simulink model "PMSM_My_PI"  (R2017b)
settings: Solver=VariableStepAuto  StartTime=0.0  StopTime=0.2  FixedStep=0.000001  MaxStep=1e-4  RelTol=1e-3
undefined symbols (not defined in the file or in its folder): sigbuilder_block
libraries: powerlib x21, simulink x1
settings Model: Creator=Linyc  LastModifiedBy=Crazyyiwen

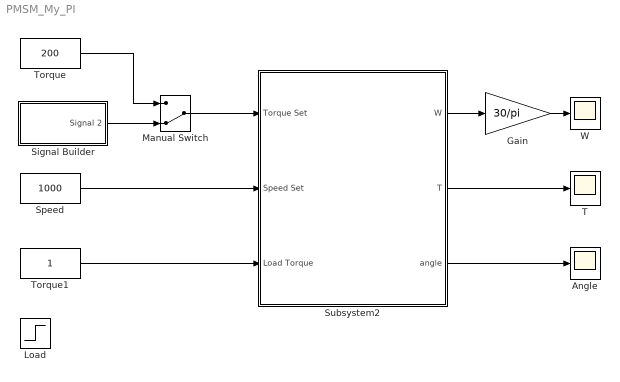
== system PMSM_My_PI ==
  Angle : Scope
  Gain : Gain  Gain=30/pi
  Load : Step  Time=0.02  After=0  SampleTime=0
  Manual Switch : ManualSwitch  CurrentSetting=0
  Signal Builder : Subsystem  Tag=STV Subsys  LoadFcn=sigbuilder_block('load');  StartFcn=sigbuilder_block('start');  StopFcn=sigbuilder_block('stop');  ClipboardFcn=sigbuilder_block('clipboard');  mask(Sigbuilder block){tuvar=[0:10]}
      mask help: Simulink:masks:SigbuilderBlock_MD
      mask init:
      | if ~strcmp(get_param(bdroot(gcbh),'SimulationStatus'),'stopped') tuvar = sigbuilder_block('maskInit'); end
      settings: CopyFcn=sigbuilder_block('copy');  DeleteFcn=sigbuilder_block('delete');  ModelCloseFcn=sigbuilder_block('modelClose');  PreSaveFcn=sigbuilder_block('preSave');  PauseFcn=sigbuilder_block('pause');  ContinueFcn=sigbuilder_block('continue');  NameChangeFcn=sigbuilder_block('namechange');  OpenFcn=sigbuilder_block('open',[424.5 166.5 847.5 399.75 ]);  CloseFcn=sigbuilder_block('close');
      mask Display: plot(0, 0, 100, 100,[2, 2, 32, 32, 2], [68, 8, 8, 68, 68],[32, 2], [38, 38], [32, 19, 2],[53, 60, 44], [32, 17, 17, 2],[16, 16, 31, 31]);txt = getActiveGroup(gcbh);text(2, 100, txt,'verticalAlignment', 'top');
  Speed : Constant  Value=1000
  Subsystem2 : Subsystem
  T : Scope
  Torque : Constant  Value=200
  Torque1 : Constant
  W : Scope
  wires:
  Speed/1 -> Subsystem2/2(Speed Set)
  Subsystem2/1(W) -> Gain/1
  Subsystem2/2(T) -> T/1
  Subsystem2/3(angle) -> Angle/1
  Gain/1 -> W/1
  Torque/1 -> Manual Switch/1
  Manual Switch/1 -> Subsystem2/1(Torque Set)
  Signal Builder/1(Signal 2) -> Manual Switch/2
  Torque1/1 -> Subsystem2/3(Load Torque)

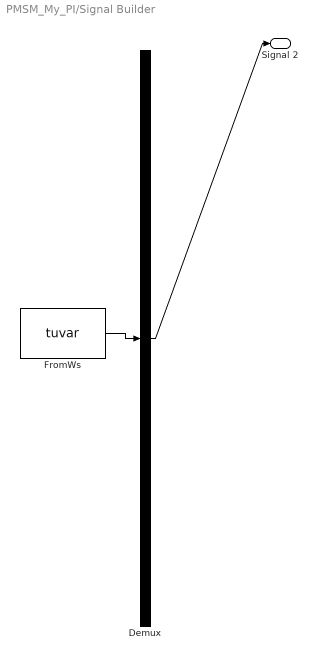
== system PMSM_My_PI/Signal Builder ==
  Demux : Demux  Tag=STV Demux  Outputs=1
  FromWs : FromWorkspace  Tag=STV FromWs  VariableName=tuvar  SampleTime=0
      SigBuilderData=|
      | common.afterFinalStr = 'Extrapolate'
      | common.sampleTime = 0
      | dataSet.timeRange = [0 2]
      | dataSet.name = 'Group 1'
      | sbobj.Groups.Name = 'Group 1'
      | sbobj.Groups.Signals.Name = 'Signal 2'
      | sbobj.Groups.Signals.XData = [0 1 1 2]
      | sbobj.Groups.Signals.YData = [200 200 0 0]
      | sbobj.Groups.TimeRange = [0 2]
  Signal 2 : Outport  Tag=STV Outport
  wires:
  FromWs/1 -> Demux/1
  Demux/1 -> Signal 2/1

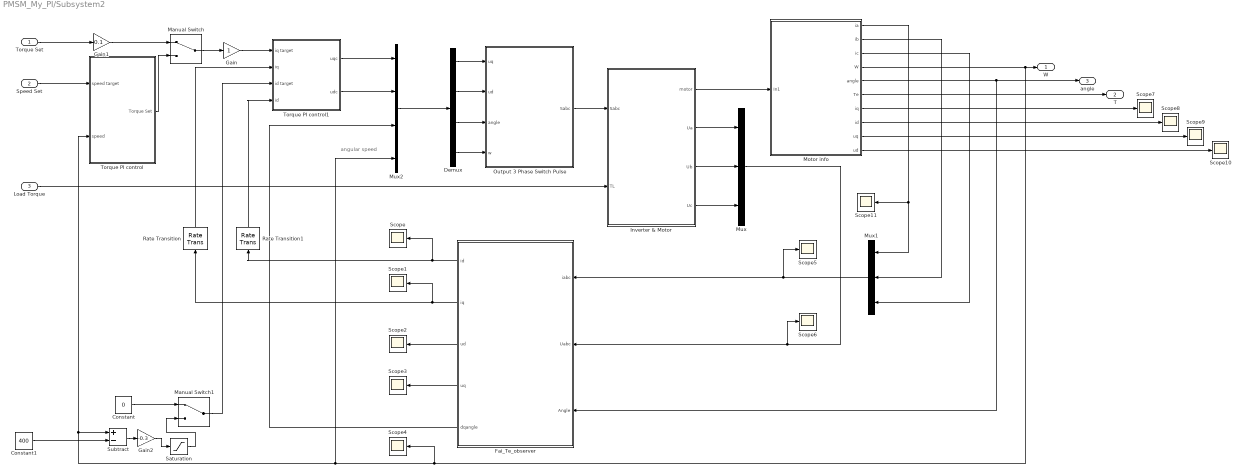
== system PMSM_My_PI/Subsystem2 ==
  note: angular speed
  Torque Set : Inport
  Speed Set : Inport  Port=2
  Load Torque : Inport  Port=3
  Constant : Constant  Value=0
  Constant1 : Constant  Value=400
  Demux : Demux
  Fai_Te_observer : Subsystem
  Gain : Gain
  Gain1 : Gain  Gain=0.1
  Gain2 : Gain  Gain=-0.3
  Inverter & Motor : Subsystem
  Manual Switch : ManualSwitch
  Manual Switch1 : ManualSwitch
  Motor info : Subsystem
  Mux : Mux  Inputs=3
  Mux1 : Mux  Inputs=3
  Mux2 : Mux
  Output 3 Phase Switch Pulse : Subsystem
  Rate Transition : RateTransition  OutPortSampleTime=0.0002
  Rate Transition1 : RateTransition  OutPortSampleTime=0.0002
  Saturation : Saturate  UpperLimit=0  LowerLimit=-150
  Scope{,1..11} (12 alike) : Scope
  Subtract : Sum  Inputs=+-
  Torque PI control : Subsystem
  Torque PI control1 : Subsystem
  W : Outport
  T : Outport  Port=2
  angle : Outport  Port=3
  wires:
  Motor info/4(W) -> Scope4/1, Mux2/4, Subtract/1, Torque PI control/2(speed), W/1
  Load Torque/1 -> Inverter & Motor/2(TL)
  Motor info/6(Te) -> T/1
  Inverter & Motor/1(motor) -> Motor info/1(In1)
  Motor info/5(angle) -> Fai_Te_observer/3(Angle), angle/1
  Motor info/1(ia) -> Scope11/1, Mux1/1
  Motor info/2(ib) -> Mux1/2
  Motor info/3(ic) -> Mux1/3
  Output 3 Phase Switch Pulse/1(Sabc) -> Inverter & Motor/1(Sabc)
  Mux1/1 -> Fai_Te_observer/1(iabc), Scope5/1
  Mux/1 -> Fai_Te_observer/2(Uabc), Scope6/1
  Mux2/1 -> Demux/1
  Motor info/7(iq) -> Scope7/1
  Motor info/8(id) -> Scope8/1
  Motor info/9(uq) -> Scope9/1
  Motor info/10(ud) -> Scope10/1
  Fai_Te_observer/1(id) -> Rate Transition1/1, Scope/1
  Fai_Te_observer/2(iq) -> Rate Transition/1, Scope1/1
  Fai_Te_observer/3(ud) -> Scope2/1
  Fai_Te_observer/4(uq) -> Scope3/1
  Speed Set/1 -> Torque PI control/1(speed target)
  Torque Set/1 -> Gain1/1
  Torque PI control/1(Torque Set) -> Manual Switch/2
  Fai_Te_observer/5(dqangle) -> Mux2/3
  Manual Switch/1 -> Gain/1
  Gain/1 -> Torque PI control1/1(iq target)
  Demux/1 -> Output 3 Phase Switch Pulse/1(uq)
  Demux/2 -> Output 3 Phase Switch Pulse/2(ud)
  Demux/3 -> Output 3 Phase Switch Pulse/3(angle)
  Torque PI control1/1(uqc) -> Mux2/1
  Rate Transition/1 -> Torque PI control1/2(iq)
  Demux/4 -> Output 3 Phase Switch Pulse/4(w)
  Gain1/1 -> Manual Switch/1
  Torque PI control1/2(udc) -> Mux2/2
  Rate Transition1/1 -> Torque PI control1/4(id)
  Constant/1 -> Manual Switch1/1
  Manual Switch1/1 -> Torque PI control1/3(id target)
  Constant1/1 -> Subtract/2
  Subtract/1 -> Gain2/1
  Gain2/1 -> Saturation/1
  Saturation/1 -> Manual Switch1/2
  Inverter & Motor/2(Ua) -> Mux/1
  Inverter & Motor/3(Ub) -> Mux/2
  Inverter & Motor/4(Uc) -> Mux/3

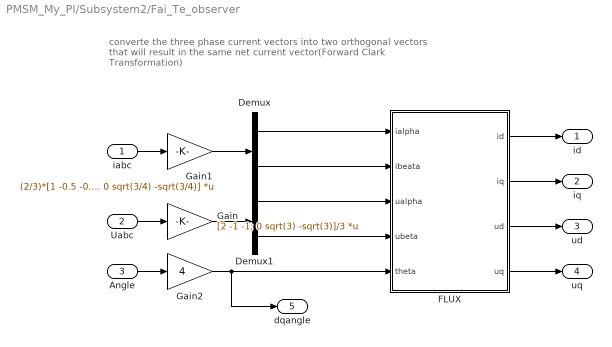
== system PMSM_My_PI/Subsystem2/Fai_Te_observer ==
  note: converte the three phase current vectors into
      | two orthogonal vectors that will result in the
      | same net current vector(Forward Clark Transformation)
  iabc : Inport
  Uabc : Inport  Port=2
  Angle : Inport  Port=3
  Demux : Demux  Outputs=2
  Demux1 : Demux  Outputs=2
  FLUX : Subsystem
  Gain : Gain  Gain=[2 -1 -1; 0 sqrt(3) -sqrt(3)]/3  Multiplication=Matrix(K*u)
  Gain1 : Gain  Gain=(2/3)*[1 -0.5 -0.5; 0 sqrt(3/4) -sqrt(3/4)]  Multiplication=Matrix(K*u)
  Gain2 : Gain  Gain=4
  id : Outport
  iq : Outport  Port=2
  ud : Outport  Port=3
  uq : Outport  Port=4
  dqangle : Outport  Port=5
  wires:
  Demux/1 -> FLUX/1(ialpha)
  Gain/1 -> Demux1/1
  iabc/1 -> Gain1/1
  Demux/2 -> FLUX/2(ibeata)
  Demux1/2 -> FLUX/4(ubeta)
  Demux1/1 -> FLUX/3(ualpha)
  Uabc/1 -> Gain/1
  Gain1/1 -> Demux/1
  Angle/1 -> Gain2/1
  Gain2/1 -> dqangle/1, FLUX/5(theta)
  FLUX/1(id) -> id/1
  FLUX/2(iq) -> iq/1
  FLUX/3(ud) -> ud/1
  FLUX/4(uq) -> uq/1

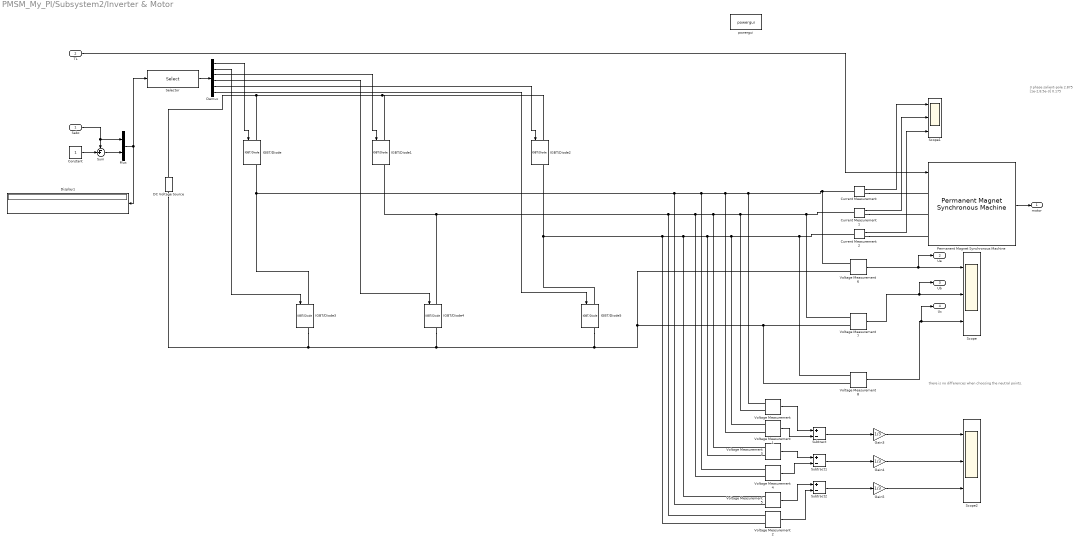
== system PMSM_My_PI/Subsystem2/Inverter & Motor ==
  note: there is no differences when choosing the neutral points.
  note: 3 phase
      | salient-pole
      |
      | 2.875
      | [1e-2,8.5e-3]
      | 0.175
  Sabc : Inport
  TL : Inport  Port=2
  Constant : Constant
  Current Measurement : powerlib/Measurements/Current Measurement  PhasorSimulation=off  OutputType=Complex  PSBequivalent=0
  Current Measurement1 : powerlib/Measurements/Current Measurement  PhasorSimulation=off  OutputType=Complex  PSBequivalent=0
  Current Measurement2 : powerlib/Measurements/Current Measurement  PhasorSimulation=off  OutputType=Complex  PSBequivalent=0
  DC Voltage Source : powerlib/Electrical Sources/DC Voltage Source  Amplitude=380  Measurements=None
  Demux : Demux  Outputs=6
  Display1 : Display
  Gain3 : Gain  Gain=1/3
  Gain4 : Gain  Gain=1/3
  Gain5 : Gain  Gain=1/3
  IGBT/Diode{,1..5} (6 alike) : powerlib/Power Electronics/IGBT//Diode  Ron=1e-2  Rs=1e4  Cs=inf  Measurements=on
  Mux : Mux  Inputs=2
  Permanent Magnet Synchronous Machine : powerlib/Machines/Permanent Magnet Synchronous Machine  NbPhases=3  FluxDistribution=Sinusoidal  RotorType=Salient-pole  MechanicalLoad=Torque Tm  PresetModel=No  ShowDetailedParameters=on  MeasurementBus=off  Resistance=2.875  Inductance=8.5e-3  dqInductances=[1e-2,8.5e-3]  La=0.000395  MachineConstant=Flux linkage established by magnets (V.s)  Flux=0.175  VoltageCst=126.966  TorqueCst=1.05  Flat=120  Mechanical=[0.0027 0.175 4 0]  PolePairs=2  InitialConditions=[0,0, 0,0]  InitialConditions5ph=[0 0 0 0 0 0]  TsPowergui=0  TsBlock=-1  RefAngle=Aligned with phase A axis (original Park)
      settings: SourceProductName=Simscape Power Systems
  Scope : Scope  NumInputPorts=3
  Scope1 : Scope  NumInputPorts=3
  Scope2 : Scope  NumInputPorts=3
  Selector : Selector  InputPortWidth=6  IndexOptions=Index vector (dialog)  Indices=[1 4 2 5 3 6]  OutputSizes=1
  Subtract : Sum  Inputs=+-
  Subtract1 : Sum  Inputs=+-
  Subtract2 : Sum  Inputs=+-
  Sum : Sum  Inputs=-+|
  Voltage Measurement{,1..8} (9 alike) : powerlib/Measurements/Voltage Measurement  PhasorSimulation=off  OutputType=Complex  PSBequivalent=0
  powergui : powerlib/powergui  Priority=1  SimulationMode=Continuous  SampleTime=0.000001  frequency=60  Iterations=50  frequencyindice=0  Pbase=100e6  ErrMax=1e-4  UnitsV=kV  UnitsW=MW  buscounter=0  FunctionMessages=on  echomessages=off  EnableUseOfTLC=off  CurrentSourceSwitches=off  DisableSnubberDevices=off  DisableRonSwitches=off  DisableVfSwitches=off  DisplayEquations=off  SolverType=Tustin/Backward Euler (TBE)  Interpol=off  ExternalGateDelay=off  methode=off  Ts=100  x0status=blocks  SPID=on  SwTol=0  HookPort=off  RestoreLinks=warning  ResistiveCurrentMeasurement=off  Frange=[0:2:500]  Ylog=off  Xlog=on  ShowGrid=off  save=off  variable=ZData  structure=0  ZoomFFT=off  StartTime=0.0  cycles=1  DisplayStyle=1  fundamental=60  FreqAxis=off  MaxFrequency=1000  frequencyindicesteady=1  RmsSteady=1  display=off
  motor : Outport
  Ua : Outport  Port=2
  Ub : Outport  Port=3
  Uc : Outport  Port=4
  wires:
  Constant/1 -> Sum/2
  Sum/1 -> Mux/2
  Mux/1 -> Display1/1, Selector/1
  TL/1 -> Permanent Magnet Synchronous Machine/1
  Permanent Magnet Synchronous Machine/1 -> motor/1
  Sabc/1 -> Mux/1, Sum/1
  Selector/1 -> Demux/1
  Demux/1 -> IGBT/Diode/1
  Demux/2 -> IGBT/Diode3/1
  Demux/3 -> IGBT/Diode1/1
  Demux/4 -> IGBT/Diode4/1
  Demux/5 -> IGBT/Diode2/1
  Demux/6 -> IGBT/Diode5/1
  Voltage Measurement7/1 -> Ub/1, Scope/2
  Voltage Measurement6/1 -> Ua/1, Scope/1
  Voltage Measurement8/1 -> Uc/1, Scope/3
  Current Measurement/1 -> Scope1/1
  Current Measurement1/1 -> Scope1/2
  Current Measurement2/1 -> Scope1/3
  Gain3/1 -> Scope2/1
  Gain4/1 -> Scope2/2
  Gain5/1 -> Scope2/3
  Voltage Measurement/1 -> Subtract/1
  Voltage Measurement1/1 -> Subtract/2
  Voltage Measurement3/1 -> Subtract1/1
  Voltage Measurement4/1 -> Subtract1/2
  Voltage Measurement5/1 -> Subtract2/1
  Voltage Measurement2/1 -> Subtract2/2
  Subtract/1 -> Gain3/1
  Subtract1/1 -> Gain4/1
  Subtract2/1 -> Gain5/1
  connections:
  IGBT/Diode/RConn1 -- Voltage Measurement5/LConn2 -- Voltage Measurement4/LConn1 -- Voltage Measurement1/LConn2 -- Voltage Measurement/LConn1 -- Voltage Measurement6/LConn1 -- Current Measurement/LConn1 -- IGBT/Diode3/LConn1
  DC Voltage Source/RConn1 -- IGBT/Diode2/LConn1 -- IGBT/Diode1/LConn1 -- IGBT/Diode/LConn1
  IGBT/Diode1/RConn1 -- Voltage Measurement2/LConn1 -- Voltage Measurement4/LConn2 -- Voltage Measurement3/LConn1 -- Voltage Measurement/LConn2 -- Voltage Measurement7/LConn1 -- Current Measurement1/LConn1 -- IGBT/Diode4/LConn1
  IGBT/Diode2/RConn1 -- Voltage Measurement2/LConn2 -- Voltage Measurement5/LConn1 -- Voltage Measurement3/LConn2 -- Voltage Measurement1/LConn1 -- Voltage Measurement8/LConn1 -- Current Measurement2/LConn1 -- IGBT/Diode5/LConn1
  IGBT/Diode5/RConn1 -- Voltage Measurement8/LConn2 -- Voltage Measurement7/LConn2 -- Voltage Measurement6/LConn2 -- DC Voltage Source/LConn1 -- IGBT/Diode3/RConn1 -- IGBT/Diode4/RConn1
  Current Measurement/RConn1 -- Permanent Magnet Synchronous Machine/LConn1
  Current Measurement1/RConn1 -- Permanent Magnet Synchronous Machine/LConn2
  Current Measurement2/RConn1 -- Permanent Magnet Synchronous Machine/LConn3

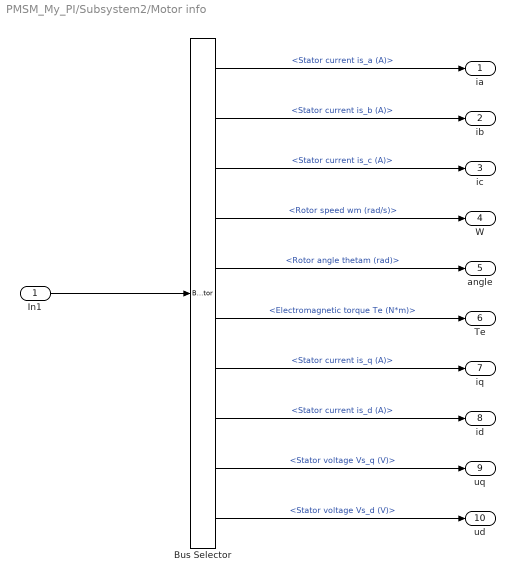
== system PMSM_My_PI/Subsystem2/Motor info ==
  In1 : Inport
  Bus Selector : BusSelector  OutputSignals=Stator current is_a (A),Stator current is_b (A),Stator current is_c (A),Rotor speed wm (rad/s),Rotor angle thetam (rad),Electromagnetic torque Te (N*m),Stator current is_q (A),Stator current is_d (A),Stator voltage Vs_q (V),Stator voltage Vs_d (V)
  ia : Outport
  ib : Outport  Port=2
  ic : Outport  Port=3
  W : Outport  Port=4
  angle : Outport  Port=5
  Te : Outport  Port=6
  iq : Outport  Port=7
  id : Outport  Port=8
  uq : Outport  Port=9
  ud : Outport  Port=10
  wires:
  In1/1 -> Bus Selector/1
  Bus Selector/2 -> ib/1  "<Stator current is_b (A)>"
  Bus Selector/3 -> ic/1  "<Stator current is_c (A)>"
  Bus Selector/6 -> Te/1  "<Electromagnetic torque Te (N*m)>"
  Bus Selector/1 -> ia/1  "<Stator current is_a (A)>"
  Bus Selector/5 -> angle/1  "<Rotor angle thetam (rad)>"
  Bus Selector/4 -> W/1  "<Rotor speed wm (rad/s)>"
  Bus Selector/7 -> iq/1  "<Stator current is_q (A)>"
  Bus Selector/8 -> id/1  "<Stator current is_d (A)>"
  Bus Selector/9 -> uq/1  "<Stator voltage Vs_q (V)>"
  Bus Selector/10 -> ud/1  "<Stator voltage Vs_d (V)>"

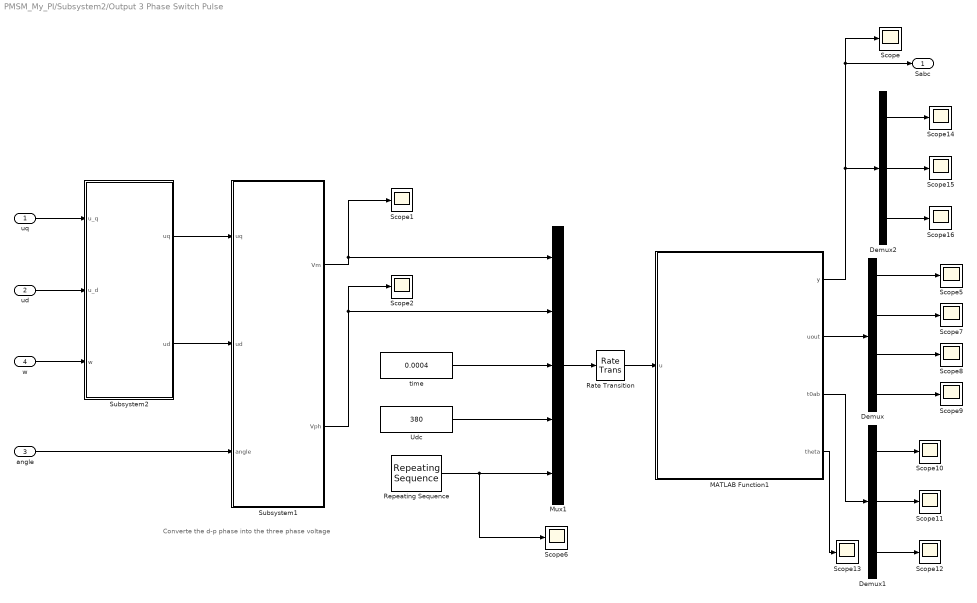
== system PMSM_My_PI/Subsystem2/Output 3 Phase Switch Pulse ==
  note: Converte the d-p phase into the three phase voltage
  uq : Inport
  ud : Inport  Port=2
  angle : Inport  Port=3
  w : Inport  Port=4
  Demux : Demux
  Demux1 : Demux  Outputs=3
  Demux2 : Demux  Outputs=3
  MATLAB Function1 : MATLAB Function  TreatAsAtomicUnit=on
  Mux1 : Mux  Inputs=5
  Rate Transition : RateTransition  OutPortSampleTime=0.000001
  Repeating Sequence : simulink/Sources/Repeating Sequence  rep_seq_t=[0 0.0002 0.0004]  rep_seq_y=[0 380 0]
  Scope{,1..2,5..16} (15 alike) : Scope
  Subsystem1 : Subsystem
  Subsystem2 : Subsystem
  Udc : Constant  Value=380
  time : Constant  Value=0.0004
  Sabc : Outport
  wires:
  time/1 -> Mux1/3
  Repeating Sequence/1 -> Scope6/1, Mux1/5
  Udc/1 -> Mux1/4
  MATLAB Function1/1(y) -> Demux2/1, Scope/1, Sabc/1
  Subsystem1/1(Vm) -> Mux1/1, Scope1/1
  Subsystem1/2(Vph) -> Mux1/2, Scope2/1
  Mux1/1 -> Rate Transition/1
  MATLAB Function1/2(uout) -> Demux/1
  Demux/4 -> Scope9/1
  Demux/2 -> Scope7/1
  Demux/3 -> Scope8/1
  Demux/1 -> Scope5/1
  MATLAB Function1/3(t0ab) -> Demux1/1
  Demux1/1 -> Scope10/1
  Demux1/3 -> Scope12/1
  Demux1/2 -> Scope11/1
  MATLAB Function1/4(theta) -> Scope13/1
  Demux2/2 -> Scope15/1
  Demux2/3 -> Scope16/1
  Demux2/1 -> Scope14/1
  Rate Transition/1 -> MATLAB Function1/1(u)
  uq/1 -> Subsystem2/1(u_q)
  ud/1 -> Subsystem2/2(u_d)
  Subsystem2/1(uq) -> Subsystem1/1(uq)
  Subsystem2/2(ud) -> Subsystem1/2(ud)
  angle/1 -> Subsystem1/3(angle)
  w/1 -> Subsystem2/3(w)

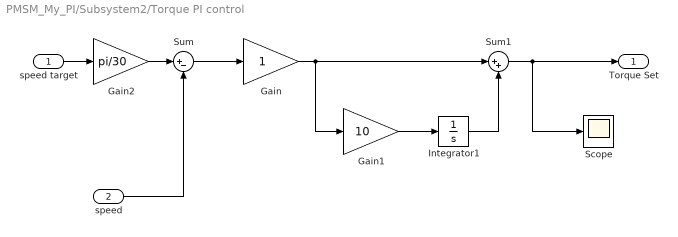
== system PMSM_My_PI/Subsystem2/Torque PI control ==
  speed target : Inport
  speed : Inport  Port=2
  Gain : Gain
  Gain1 : Gain  Gain=10
  Gain2 : Gain  Gain=pi/30
  Integrator1 : Integrator
  Scope : Scope
  Sum : Sum  Inputs=|+-
  Sum1 : Sum  Inputs=|++
  Torque Set : Outport
  wires:
  speed target/1 -> Gain2/1
  Sum/1 -> Gain/1
  speed/1 -> Sum/2
  Gain2/1 -> Sum/1
  Gain/1 -> Gain1/1, Sum1/1
  Integrator1/1 -> Sum1/2
  Sum1/1 -> Scope/1, Torque Set/1
  Gain1/1 -> Integrator1/1

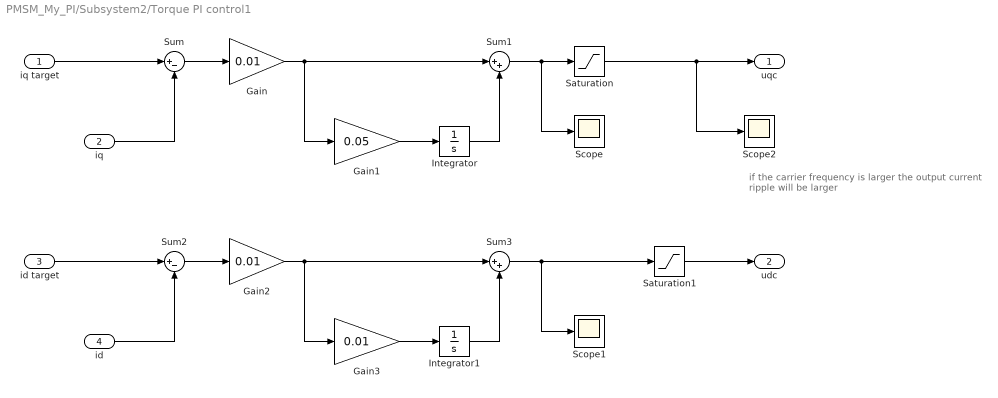
== system PMSM_My_PI/Subsystem2/Torque PI control1 ==
  note: if the carrier frequency is larger the
      | output current ripple will be larger
  iq target : Inport
  iq : Inport  Port=2
  id target : Inport  Port=3
  id : Inport  Port=4
  Gain : Gain  Gain=0.01
  Gain1 : Gain  Gain=0.05
  Gain2 : Gain  Gain=0.01
  Gain3 : Gain  Gain=0.01
  Integrator : Integrator
  Integrator1 : Integrator
  Saturation : Saturate  UpperLimit=1  LowerLimit=-1
  Saturation1 : Saturate  UpperLimit=1  LowerLimit=-1
  Scope : Scope
  Scope1 : Scope
  Scope2 : Scope
  Sum : Sum  Inputs=|+-
  Sum1 : Sum  Inputs=|++
  Sum2 : Sum  Inputs=|+-
  Sum3 : Sum  Inputs=|++
  uqc : Outport
  udc : Outport  Port=2
  wires:
  Gain1/1 -> Integrator/1
  Integrator/1 -> Sum1/2
  Gain/1 -> Gain1/1, Sum1/1
  iq/1 -> Sum/2
  Sum/1 -> Gain/1
  id target/1 -> Sum2/1
  Sum2/1 -> Gain2/1
  id/1 -> Sum2/2
  Gain2/1 -> Sum3/1, Gain3/1
  Sum3/1 -> Saturation1/1, Scope1/1
  Integrator1/1 -> Sum3/2
  Gain3/1 -> Integrator1/1
  Saturation1/1 -> udc/1
  iq target/1 -> Sum/1
  Sum1/1 -> Saturation/1, Scope/1
  Saturation/1 -> Scope2/1, uqc/1

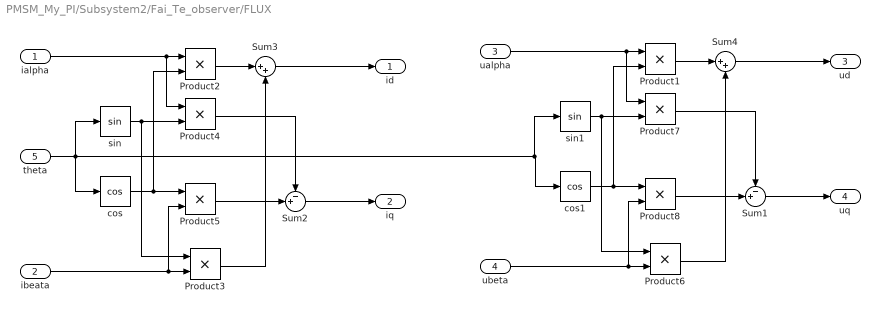
== system PMSM_My_PI/Subsystem2/Fai_Te_observer/FLUX ==
  ialpha : Inport
  ibeata : Inport  Port=2
  ualpha : Inport  Port=3
  ubeta : Inport  Port=4
  theta : Inport  Port=5
  Product{1..8} (8 alike) : Product
  Sum1 : Sum  Inputs=-+|
  Sum2 : Sum  Inputs=-+|
  Sum3 : Sum  Inputs=|++
  Sum4 : Sum  Inputs=|++
  cos : Trigonometry  Operator=cos
  cos1 : Trigonometry  Operator=cos
  sin : Trigonometry
  sin1 : Trigonometry
  id : Outport
  iq : Outport  Port=2
  ud : Outport  Port=3
  uq : Outport  Port=4
  wires:
  ialpha/1 -> Product4/1, Product2/1
  cos/1 -> Product5/1, Product2/2
  ibeata/1 -> Product5/2, Product3/2
  sin/1 -> Product4/2, Product3/1
  Product2/1 -> Sum3/1
  Product3/1 -> Sum3/2
  Product4/1 -> Sum2/1
  Product5/1 -> Sum2/2
  Sum3/1 -> id/1
  Sum2/1 -> iq/1
  Sum1/1 -> uq/1
  Sum4/1 -> ud/1
  Product8/1 -> Sum1/2
  Product7/1 -> Sum1/1
  Product6/1 -> Sum4/2
  Product1/1 -> Sum4/1
  sin1/1 -> Product6/1, Product7/2
  ubeta/1 -> Product6/2, Product8/2
  cos1/1 -> Product1/2, Product8/1
  ualpha/1 -> Product1/1, Product7/1
  theta/1 -> sin1/1, cos1/1, sin/1, cos/1

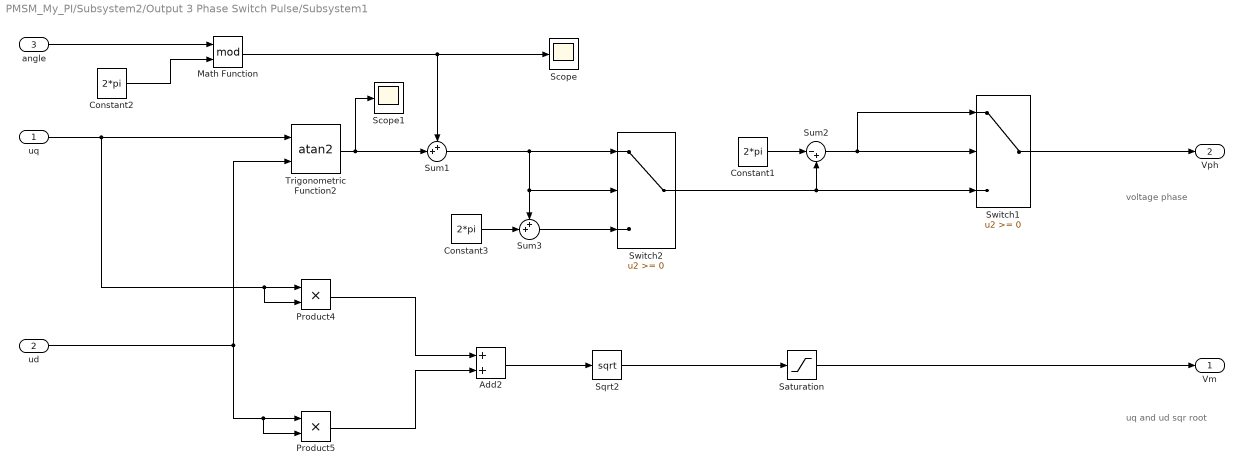
== system PMSM_My_PI/Subsystem2/Output 3 Phase Switch Pulse/Subsystem1 ==
  note: voltage phase
  note: uq and ud sqr root
  uq : Inport
  ud : Inport  Port=2
  angle : Inport  Port=3
  Add2 : Sum
  Constant1 : Constant  Value=2*pi
  Constant2 : Constant  Value=2*pi
  Constant3 : Constant  Value=2*pi
  Math Function : Math  Operator=mod  SaturateOnIntegerOverflow=on
  Product4 : Product
  Product5 : Product
  Saturation : Saturate  UpperLimit=380  LowerLimit=0
  Scope : Scope
  Scope1 : Scope
  Sqrt2 : Sqrt  SaturateOnIntegerOverflow=on
  Sum1 : Sum  Inputs=++|
  Sum2 : Sum  Inputs=|-+
  Sum3 : Sum  Inputs=++|
  Switch1 : Switch
  Switch2 : Switch
  Trigonometric Function2 : Trigonometry  Operator=atan2
  Vm : Outport
  Vph : Outport  Port=2
  wires:
  Product5/1 -> Add2/2
  ud/1 -> Trigonometric Function2/2, Product5/2, Product5/1
  Sqrt2/1 -> Saturation/1
  Product4/1 -> Add2/1
  Add2/1 -> Sqrt2/1
  uq/1 -> Trigonometric Function2/1, Product4/2, Product4/1
  Sum3/1 -> Switch2/3
  Sum1/1 -> Sum3/1, Switch2/2, Switch2/1
  Constant3/1 -> Sum3/2
  Trigonometric Function2/1 -> Scope1/1, Sum1/2
  Sum2/1 -> Switch1/2, Switch1/1
  Constant1/1 -> Sum2/1
  Switch2/1 -> Switch1/3, Sum2/2
  Switch1/1 -> Vph/1
  angle/1 -> Math Function/1
  Constant2/1 -> Math Function/2
  Math Function/1 -> Scope/1, Sum1/1
  Saturation/1 -> Vm/1

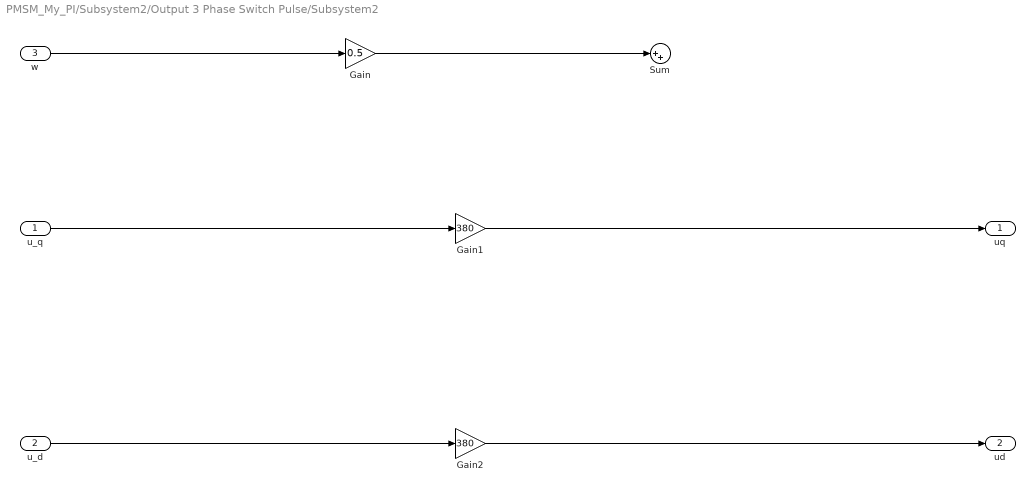
== system PMSM_My_PI/Subsystem2/Output 3 Phase Switch Pulse/Subsystem2 ==
  u_q : Inport
  u_d : Inport  Port=2
  w : Inport  Port=3
  Gain : Gain  Gain=0.5
  Gain1 : Gain  Gain=380
  Gain2 : Gain  Gain=380
  Sum : Sum  Inputs=|++
  uq : Outport
  ud : Outport  Port=2
  wires:
  u_d/1 -> Gain2/1
  w/1 -> Gain/1
  Gain/1 -> Sum/1
  u_q/1 -> Gain1/1
  Gain1/1 -> uq/1
  Gain2/1 -> ud/1

== matlab function PMSM_My_PI/Subsystem2/Output 3 Phase Switch Pulse/MATLAB Function1 ==
  data: u input size=5; y output; uout output; t0ab output; theta output
function [y, uout, t0ab,theta] = svpwm005(u)
Vm=u(1);
ph=u(2);
tp=u(3);
Udc=u(4);
du=pi/3;

% define 8 vectors
u0=[0 0 0];
u1=[0 0 1];
u2=[0 1 0];
u3=[0 1 1];
u4=[1 0 0];
u5=[1 0 1];
u6=[1 1 0];
u7=[1 1 1];

% determine which sector ph belongs to
if ph>0 && ph<=du
    theta=ph;
    h=1;
    ua=u4;
    ub=u6;
elseif ph>du && ph<=2*du
    theta=2*du-ph;
    h=2;
    ua=u2;
    ub=u6;
elseif ph>2*du && ph<=3*du
    theta=ph-2*du;
    h=3;
    ua=u2;
    ub=u3;
elseif ph>3*du && ph<=4*du
    theta=4*du-ph;
    h=4;
    ua=u1;
    ub=u3;
elseif ph>4*du && ph<=5*du
    theta=ph-4*du;
    h=5;
    ua=u1;
    ub=u5;
else
    theta=6*du-ph;
    h=6;
    ua=u4;
    ub=u5;
end

% calculate ta,tb,tc
ta=1.5*(cos(theta)-1/sqrt(3)*sin(theta))*Vm*tp/Udc;
tb=sqrt(3)*Vm*sin(theta)*tp/Udc;
t0=tp-ta-tb;
if t0<0
    ta=ta/(ta+tb)*tp;
    tb=tp-ta;
    t0=0;
end
% transfor the time into the voltage
usw1=Udc*t0/tp/2;
usw2=Udc*ta/tp+usw1;
usw3=Udc*tb/tp+usw2;
%判断并输出
if u(5)>=0 && u(5)<usw1
    y=u0;
elseif u(5)>=usw1 && u(5)<usw2
    y=ua;
elseif u(5)>=usw2 && u(5)<usw3
    y=ub;
else
    y=u7;
end
uout=[usw1 usw2 usw3 u(5)];
t0ab=[t0 ta tb];
